simulink model "sampleModel1698_4"  (R2023a)
settings: Solver=VariableStepAuto  StartTime=0.0  StopTime=10.0  RelTol=1e-3
libraries: hdlsllib x1, simulink x1
settings Model: Creator=user1  LastModifiedBy=user1

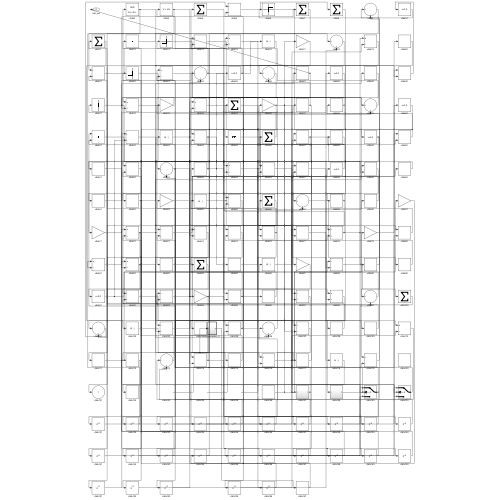
[thumbnail: Simulink's stored preview of the top-level diagram]
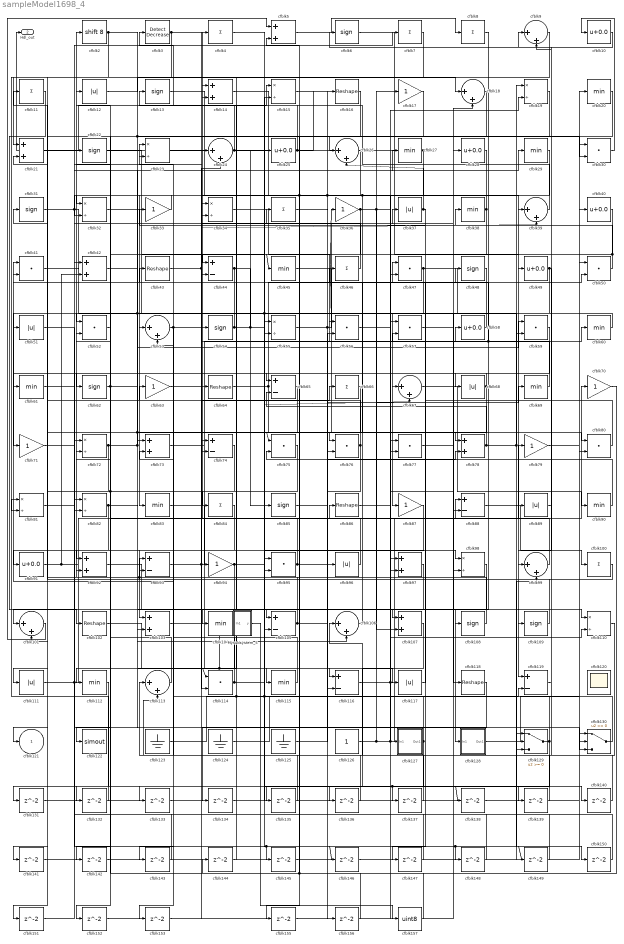
== system sampleModel1698_4 ==
  Mysubsystem_5 : Subsystem  TreatAsAtomicUnit=on  RTWFcnName=Mysubsystem_5
      settings: RTWFcnNameOpts=User specified  RTWFileNameOpts=Use function name
  cfblk{10,25,28,40,49,58,91} (7 alike) : Bias  Bias=0.0  SaturateOnIntegerOverflow=off
  cfblk{4,7..8,11,35,46,66,84,100} (9 alike) : Sum  Inputs=+  OutDataTypeStr=uint8
  cfblk{9,18,24,26,39,53,67,99,101,106,113} (11 alike) : Sum  Inputs=|++  OutDataTypeStr=uint8
  cfblk{16,43,64,86,102,118} (6 alike) : Reshape
  cfblk{5,14,21,42,73,78,92,97,103,107} (10 alike) : Sum  OutDataTypeStr=uint8
  cfblk{20,27,29,38,45,60..61,69,83,90,104,112,115} (13 alike) : MinMax  OutDataTypeStr=uint8
  cfblk{44,65,74,88,93,105,116,119} (8 alike) : Sum  Inputs=+-  OutDataTypeStr=uint8
  cfblk{6,13,22,31,48,54,62,85,108..109} (10 alike) : Signum
  cfblk{15,19,23,32,34,55,72,81..82,98,110} (11 alike) : Product  Inputs=*/  OutDataTypeStr=uint8  RndMeth=Zero  SaturateOnIntegerOverflow=on
  cfblk{12,37,51,68,89,96,111,117} (8 alike) : Abs  OutDataTypeStr=uint8  SaturateOnIntegerOverflow=off
  cfblk{30,41,47,50,52,56..57,59,75..77,80,95,114} (14 alike) : DotProduct  OutDataTypeStr=uint8
  cfblk120 : Scope
      settings: Floating=on
  cfblk122 : ToWorkspace  VariableName=simout  SaveFormat=Timeseries  SampleTime=-1
  cfblk123 : Ground
  cfblk124 : Ground
  cfblk125 : Ground
  cfblk126 : Constant  OutDataTypeStr=uint8  SampleTime=-1
  cfblk127 : Subsystem
      settings: LibrarySourceBlock=|
      | hdlsllib/Ports &
      | Subsystems/Subsystem
  cfblk128 : Subsystem
      settings: LibrarySourceBlock=|
      | hdlsllib/Ports &
      | Subsystems/Subsystem
  cfblk129 : Switch  OutDataTypeStr=uint8  SaturateOnIntegerOverflow=off  InputSameDT=off
  cfblk130 : Switch  OutDataTypeStr=uint8  SaturateOnIntegerOverflow=off  InputSameDT=off
  cfblk{131..153,155..156} (25 alike) : Delay  SampleTime=1
  cfblk157 : DataTypeConversion  OutDataTypeStr=uint8  SaturateOnIntegerOverflow=off  RndMeth=Floor
  cfblk{17,33,36,63,70..71,79,87,94} (9 alike) : Gain  OutDataTypeStr=uint8
  cfblk2 : ArithShift  BitShiftNumber=8
  cfblk3 : simulink/Logic and Bit Operations/Detect Decrease  vinit=0.0  OutDataTypeStr=uint8
      settings: LibrarySourceBlock=|
      | hdlsllib/Logic and Bit
      | Operations/Detect
      | Decrease
  cfblk121 : Outport  OutDataTypeStr=uint8  VectorParamsAs1DForOutWhenUnconnected=off
  Hdl_out : Outport  Port=2  OutDataTypeStr=uint8
  wires:
  cfblk39/1 -> cfblk13/1
  cfblk49/1 -> cfblk87/1, cfblk99/1
  cfblk119/1 -> cfblk38/1
  cfblk105/1 -> cfblk2/1, cfblk78/2
  cfblk5/1 -> cfblk8/1
  cfblk10/1 -> cfblk6/1
  cfblk130/1 -> cfblk41/1
  cfblk102/1 -> cfblk115/1
  cfblk7/1 -> cfblk91/1
  cfblk38/1 -> cfblk83/1, cfblk147/1
  cfblk111/1 -> cfblk86/1, cfblk130/3
  cfblk123/1 -> cfblk77/1, cfblk15/2
  cfblk11/1 -> cfblk102/1
  cfblk17/1 -> cfblk26/1
  cfblk60/1 -> cfblk52/1
  cfblk117/1 -> cfblk47/1
  cfblk116/1 -> cfblk70/1, cfblk19/2
  cfblk69/1 -> cfblk36/1, cfblk48/1
  cfblk24/1 -> cfblk59/2, cfblk67/2, cfblk3/1
  cfblk127/1(Out1) -> cfblk53/2, cfblk132/1
  cfblk30/1 -> cfblk10/1
  cfblk45/1 -> cfblk80/1
  cfblk44/1 -> cfblk71/1, cfblk85/1
  cfblk50/1 -> cfblk45/1, cfblk33/1
  cfblk126/1 -> cfblk88/1, cfblk110/2, cfblk17/1
  cfblk64/1 -> cfblk50/2, cfblk97/1
  cfblk72/1 -> cfblk129/2, cfblk29/1, cfblk121/1
  cfblk6/1 -> cfblk119/1
  cfblk85/1 -> cfblk69/1
  cfblk87/1 -> cfblk103/1
  cfblk83/1 -> cfblk116/1
  cfblk73/1 -> cfblk60/1
  cfblk74/1 -> cfblk122/1, cfblk82/2
  cfblk95/1 -> cfblk4/1, cfblk140/1
  cfblk101/1 -> cfblk5/1
  cfblk108/1 -> cfblk93/1, cfblk21/2
  cfblk80/1 -> cfblk54/1
  cfblk2/1 -> cfblk117/1, cfblk75/1, cfblk30/2, cfblk21/1
  cfblk114/1 -> cfblk148/1, cfblk149/1, cfblk23/1
  cfblk54/1 -> cfblk25/1, cfblk97/2, cfblk53/1
  cfblk91/1 -> cfblk79/1, cfblk42/2
  cfblk19/1 -> cfblk51/1
  cfblk22/1 -> cfblk96/1
  cfblk94/1 -> cfblk137/1, cfblk138/1, cfblk101/1
  cfblk40/1 -> cfblk62/1
  cfblk93/1 -> cfblk57/2, cfblk66/1
  cfblk124/1 -> cfblk119/2
  cfblk29/1 -> Mysubsystem_5/1(In1), cfblk114/1, cfblk65/1
  cfblk96/1 -> cfblk72/2
  cfblk86/1 -> cfblk58/1
  cfblk53/1 -> cfblk77/2, cfblk133/1
  cfblk99/1 -> cfblk43/1
  cfblk32/1 -> cfblk55/1
  cfblk18/1 -> cfblk105/1
  cfblk110/1 -> cfblk113/2
  cfblk67/1 -> cfblk90/1
  cfblk55/1 -> cfblk28/1, cfblk78/1
  cfblk92/1 -> cfblk128/1(In1)
  cfblk20/1 -> cfblk108/1
  cfblk12/1 -> cfblk18/1
  cfblk62/1 -> cfblk112/1, cfblk59/1
  cfblk79/1 -> cfblk40/1
  cfblk128/1(Out1) -> cfblk20/1
  cfblk56/1 -> cfblk130/2
  cfblk23/1 -> cfblk127/1(In1)
  cfblk13/1 -> cfblk95/1
  cfblk109/1 -> cfblk31/1
  cfblk37/1 -> cfblk26/2, cfblk67/1
  cfblk41/1 -> cfblk73/1, cfblk55/2
  cfblk71/1 -> cfblk24/1
  cfblk43/1 -> cfblk94/1, cfblk39/2
  cfblk3/1 -> cfblk81/2, cfblk39/1
  cfblk52/1 -> cfblk92/1
  cfblk77/1 -> cfblk118/1
  cfblk34/1 -> cfblk56/1
  cfblk33/1 -> cfblk32/1
  cfblk115/1 -> cfblk63/1
  cfblk9/1 -> cfblk44/1
  cfblk68/1 -> cfblk95/2, cfblk61/1
  cfblk90/1 -> cfblk35/1
  cfblk27/1 -> cfblk76/1, cfblk32/2, Hdl_out/1
  cfblk42/1 -> cfblk109/1
  cfblk59/1 -> cfblk104/1
  cfblk35/1 -> cfblk98/1
  cfblk125/1 -> cfblk56/2
  cfblk14/1 -> cfblk49/1
  cfblk89/1 -> cfblk9/1
  cfblk21/1 -> cfblk15/1
  cfblk100/1 -> cfblk93/2
  cfblk51/1 -> cfblk145/1, cfblk146/1
  cfblk81/1 -> cfblk37/1
  cfblk76/1 -> cfblk116/2, cfblk11/1
  cfblk31/1 -> cfblk98/2, cfblk27/1
  cfblk36/1 -> cfblk88/2, cfblk107/2, cfblk84/1
  cfblk58/1 -> cfblk14/1
  cfblk82/1 -> cfblk106/2, cfblk131/1
  cfblk63/1 -> cfblk30/1
  cfblk26/1 -> cfblk74/2
  cfblk75/1 -> cfblk103/2
  cfblk129/1 -> cfblk23/2, cfblk64/1, cfblk135/1
  cfblk28/1 -> cfblk76/2, cfblk114/2
  cfblk61/1 -> cfblk7/1
  cfblk88/1 -> cfblk100/1
  cfblk106/1 -> cfblk46/1
  cfblk103/1 -> cfblk107/1
  cfblk47/1 -> cfblk89/1, cfblk101/2
  cfblk46/1 -> cfblk34/2
  cfblk8/1 -> cfblk68/1
  cfblk25/1 -> cfblk14/2, cfblk16/1
  cfblk57/1 -> cfblk110/1
  cfblk78/1 -> cfblk19/1, cfblk150/1, cfblk65/2
  cfblk48/1 -> cfblk41/2
  cfblk84/1 -> cfblk111/1
  cfblk113/1 -> cfblk22/1
  cfblk131/1 -> cfblk105/2
  cfblk132/1 -> cfblk81/1
  cfblk133/1 -> cfblk47/2
  cfblk118/1 -> cfblk134/1
  cfblk134/1 -> cfblk130/1
  cfblk135/1 -> cfblk73/2
  cfblk107/1 -> cfblk136/1
  cfblk136/1 -> cfblk34/1
  cfblk137/1 -> cfblk113/1
  cfblk138/1 -> cfblk99/2
  cfblk4/1 -> cfblk139/1
  cfblk139/1 -> cfblk106/1
  cfblk140/1 -> cfblk9/2
  cfblk112/1 -> cfblk141/1
  cfblk141/1 -> cfblk80/2
  cfblk104/1 -> cfblk142/1
  cfblk142/1 -> cfblk50/1
  cfblk98/1 -> cfblk143/1
  cfblk143/1 -> cfblk82/1
  cfblk70/1 -> cfblk144/1
  cfblk144/1 -> cfblk44/2
  cfblk145/1 -> cfblk129/1
  cfblk146/1 -> cfblk129/3
  cfblk147/1 -> cfblk5/2
  cfblk148/1 -> cfblk52/2
  cfblk149/1 -> cfblk42/1
  cfblk150/1 -> cfblk92/2
  cfblk65/1 -> cfblk151/1
  cfblk151/1 -> cfblk72/1
  cfblk16/1 -> cfblk152/1
  cfblk152/1 -> cfblk24/2
  cfblk97/1 -> cfblk153/1
  cfblk153/1 -> cfblk57/1
  cfblk66/1 -> cfblk155/1
  cfblk155/1 -> cfblk18/2
  cfblk15/1 -> cfblk156/1
  cfblk156/1 -> cfblk74/1
  cfblk157/1 -> cfblk75/2, cfblk12/1
  Mysubsystem_5/1(y) -> cfblk157/1

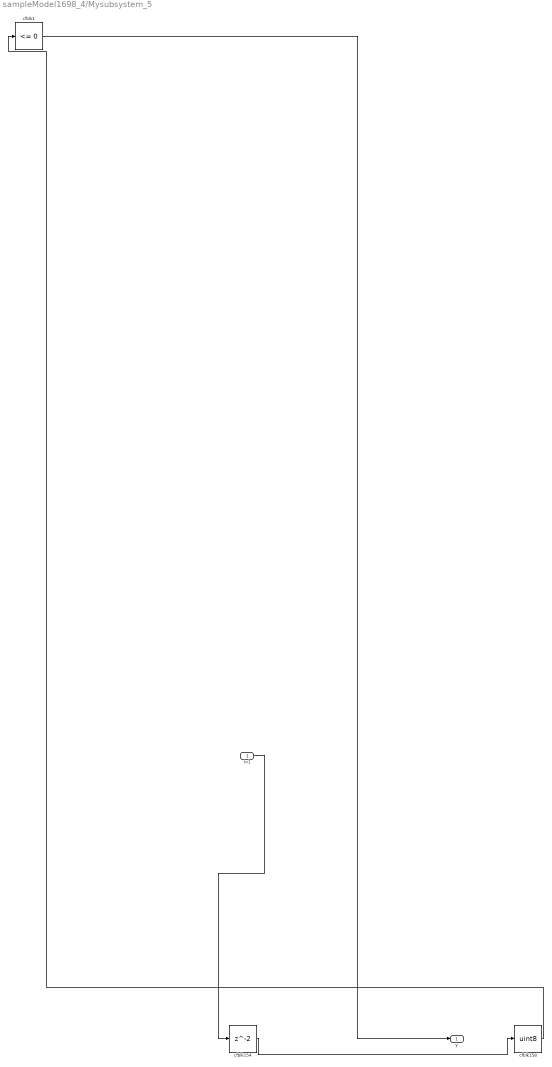
== system sampleModel1698_4/Mysubsystem_5 ==
  In1 : Inport
  cfblk1 : hdlsllib/Logic and Bit Operations/Compare To Zero  relop=<=  OutDataTypeStr=boolean
  cfblk154 : Delay  SampleTime=1
  cfblk158 : DataTypeConversion  OutDataTypeStr=uint8  SaturateOnIntegerOverflow=off  RndMeth=Floor
  y : Outport
  wires:
  cfblk1/1 -> y/1
  cfblk154/1 -> cfblk158/1
  In1/1 -> cfblk154/1
  cfblk158/1 -> cfblk1/1

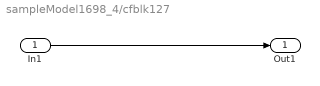
== system sampleModel1698_4/cfblk127 ==
  In1 : Inport
  Out1 : Outport
  wires:
  In1/1 -> Out1/1

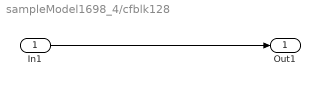
== system sampleModel1698_4/cfblk128 ==
  In1 : Inport
  Out1 : Outport
  wires:
  In1/1 -> Out1/1
